simulink model "Speedgoat_Standalone_Sim_Dyno"  (R2021a)
settings: Solver=FixedStepDiscrete  StartTime=0.0  StopTime=inf  FixedStep=ModelTs  RelTol=1e-3
PreLoadFcn:
  | clc;
  | clear;
  | addpath ../
  | addpath(genpath('../../../settings/ParametersFiles/'))
  | addpath(genpath('../../../source/simulink/'))
  | BusInit;
  | filename_motor='';
  | filename_board='';
  | Thermal.Trotor = 25;
  | Thermal.Tstator = 25;
  | adc_out_mode = 1;  % 'ADC_voltage'  -- 0 --> 'ADC_counts'
  | InputCircuit.Vr = 230;  % ac voltage
  | ModelTs = 62.5e-6;  % 16KHz
undefined symbols (not defined in the file or in its folder): IO316, IO3xx, Motor
libraries: speedgoatlib_IO142 x3, speedgoatlib_fpga_pwm x3, simulink_extras x1, MapleSim_bpm_dq_dyno_xi_ie_16k_2018a x1, speedgoatlib_fpga x1
settings Model: SimulationMode=external  Creator=BEATOA  LastModifiedBy=lab.motori2
settings SolverCC: ConcurrentTasks=on  AlgebraicLoopSolver=TrustRegion  PositivePriorityOrder=on
settings DataIOCC: ReturnWorkspaceOutputs=off
settings OptimizationCC: BlockReduction=off  OptimizeBlockIOStorage=off
settings DebuggingCC: TasksWithSamePriorityMsg=none  SFMachineParentedDataDiag=warning  ArithmeticOperatorsInVariantConditions=warning
settings HardwareCC: ProdBitPerLong=64  ProdLongLongMode=on  ProdHWDeviceType=Intel->x86-64 (Linux 64)
settings SFSimCC: SimUseLocalCustomCode=off  CustomCodeUndefinedFunction=UseInterfaceOnly
settings RTWCC: Description=Simulink Real-Time  SystemTargetFile=slrealtime.tlc  TemplateMakefile=slrealtime_default_tmf  RTWUseLocalCustomCode=off  Toolchain=Simulink Real-Time Toolchain  BuildConfiguration=Faster Runs  CodeExecutionProfiling=on  TargetLang=C++

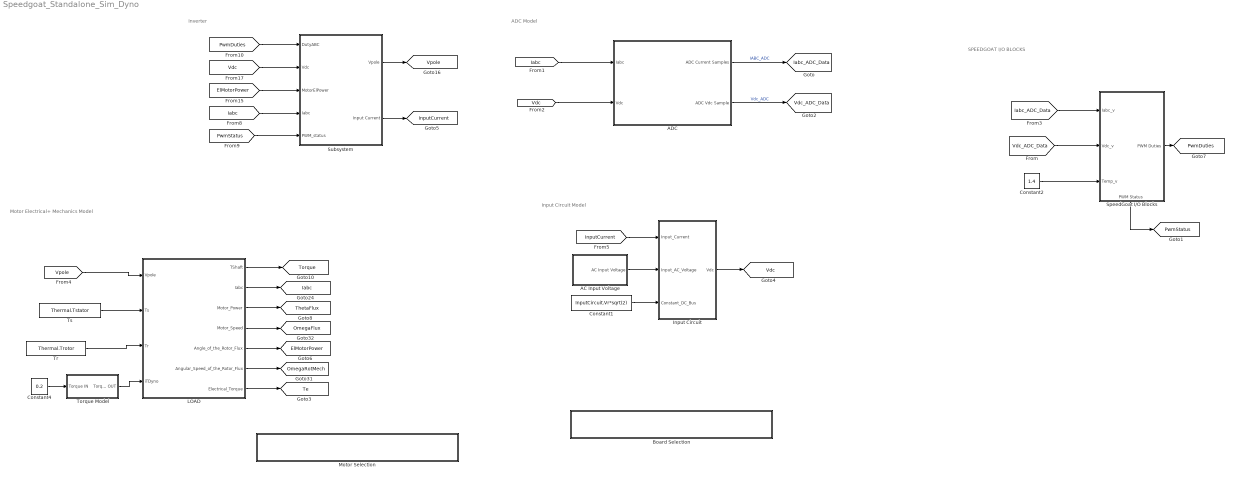
== system Speedgoat_Standalone_Sim_Dyno ==
  note: Inverter
  note: ADC Model
  note: Motor Electrical+ Mechanics Model
  note: SPEEDGOAT I/O BLOCKS
  note: Input Circuit Model
  AC Input Voltage : Subsystem
  ADC : Subsystem  mask{C1=InputCircuit.C1, C2=InputCircuit.C2, Cvolt=InputCircuit.Cvolt, ADCBit=InputCircuit.ADCBit, Vcc=InputCircuit.Vcc}
  Board Selection : Subsystem  TreatAsAtomicUnit=on  mask{ParamsFile=ColoradoPreliminary_AC230VPFC.xml}
      mask prompts: ParamsFile "Motor Parameters Selection"
      mask init:
      | myVal = evalin('base','filename_board');
      | set_param(gcb,'ParamsFile',myVal);
      settings: OpenFcn=|
      | filename_board = uigetfile({'*.xml'}, 'Select a board parameters File', ...
      |     '../../../settings/ParametersFiles/Rectifier_Parameters/');
      | run_rect_xml(filename_board);
      | set_param(gcb,'ParamsFile',filename_board);
      mask Display: disp(get_param(gcb,'ParamsFile'));
  Constant1 : Constant  Value=InputCircuit.Vr*sqrt(2)
  Constant2 : Constant  Value=1.4
  Constant4 : Constant  Value=0.2
  Input Circuit : Subsystem  Variant=on  VariantControlMode=label  VariantControl=Choice  LabelModeActiveChoice=Choice_2
  LOAD : Subsystem  Variant=on  VariantControlMode=label  LabelModeActiveChoice=Complete Motor
  Motor Selection : Subsystem  TreatAsAtomicUnit=on  mask{ParamsFile=BPM_Hefei_H27.xml}
      mask prompts: ParamsFile "Motor Parameters Selection"
      mask init:
      | myVal = evalin('base','filename_motor');
      | set_param(gcb,'ParamsFile',myVal);
      settings: OpenFcn=|
      | filename_motor = uigetfile({'*.xml'}, 'Select a motor parameters File', ...
      |     '../../../settings/ParametersFiles/Motor_Parameters/');
      | run_motor_bpm_xml(filename_motor);
      | set_param(gcb,'ParamsFile',filename_motor);
      mask Display: disp(get_param(gcb,'ParamsFile'));
  SpeedGoat I/O Blocks : Subsystem
      settings: PortSchema="{\"entries\":[{\"content\":{\"sides\":[{\"content\":{\"connectorIds\":[\"In1\",\"In2\",\"In3\"]},\"type\":\"ConnectorPlacement.EquallySpacedRectSide\",\"uuid\":\"6b9aa341-3ac4-4bf9-8aae-3ce5ce9c7d2d\"},{\"content\":{\"connectorIds\":[\"Out1\"],\"side\":\"RIGHT\"},\"type\":\"ConnectorPlacement.EquallySpacedRectSide\",\"uuid\":\"0e7969fa-09d9-4686-a5e1-30592a058991\"},{\"content\":{\"connectorIds\":[],\"side\":\"TOP\"},\"type\":\"ConnectorPlacement.EquallySpacedRectSide\",\"uuid\":\"94aad33f-2d4e-4106-b9bf-df6b0e16ba85\"},{\"content\":{\"connectorIds\":[\"Out2\"],\"side\":\"BOTTOM\"},\"type\":\"ConnectorPlacement.EquallySpacedRectSide\",\"uuid\":\"230b77cf-a16b-4a04-9d46-02ae57ab6957\"}]},\"type\":\"ConnectorPlacement.EquallySpacedConnector\",\"uuid\":\"7bdcd0a4-d700-4dbb-82d4-1eb3a47212ed\"}],\"packageUris\":[\"http://schema.mathworks.com/mf0/Connector/R2020b\"],\"version\":\"1.0\"}"
  Subsystem : Subsystem
  Torque Model : Subsystem
  Tr : Constant  Value=Thermal.Trotor
  Ts : Constant  Value=Thermal.Tstator
  tag scope: ElMotorPower=global, Iabc=global, Iabc_ADC_Data=global, InputCurrent=global, OmegaFlux=global, OmegaRotMech=global, PwmDuties=global, PwmStatus=global, Te=global, ThetaFlux=global, Torque=global, Vdc=global, Vdc_ADC_Data=global, Vpole=global
  wires:
  [Vdc] -> ADC/2(Vdc)
  ADC/1(ADC Current Samples) -> [Iabc_ADC_Data]  "IABC_ADC"
  ADC/2(ADC Vdc Sample) -> [Vdc_ADC_Data]  "Vdc_ADC"
  [Iabc] -> ADC/1(Iabc)
  [PwmDuties] -> Subsystem/1(DutyABC)
  [Vdc] -> Subsystem/2(Vdc)
  [ElMotorPower] -> Subsystem/3(MotorElPower)
  [Iabc] -> Subsystem/4(Iabc)
  [PwmStatus] -> Subsystem/5(PWM_status)
  Subsystem/1("Vpole ") -> [Vpole]
  Subsystem/2(Input Current) -> [InputCurrent]
  [Vpole] -> LOAD/1(Vpole)
  Ts/1 -> LOAD/2(Ts)
  Tr/1 -> LOAD/3(Tr)
  LOAD/1(TShaft) -> [Torque]
  LOAD/2(Iabc) -> [Iabc]
  LOAD/3(Motor_Power) -> [ThetaFlux]
  LOAD/4(Motor_Speed) -> [OmegaFlux]
  LOAD/5(Angle_of_the_Rotor_Flux) -> [ElMotorPower]
  LOAD/6(Angular_Speed_of_the_Rotor_Flux) -> [OmegaRotMech]
  LOAD/7(Electrical_Torque) -> [Te]
  Torque Model/1(Torque OUT) -> LOAD/4(iTDyno)
  [InputCurrent] -> Input Circuit/1(Input_Current)
  AC Input Voltage/1(AC Input Voltage) -> Input Circuit/2(Input_AC_Voltage)
  Constant1/1 -> Input Circuit/3(Constant_DC_Bus)
  Input Circuit/1(Vdc) -> [Vdc]
  [Iabc_ADC_Data] -> SpeedGoat I/O Blocks/1(Iabc_v)
  [Vdc_ADC_Data] -> SpeedGoat I/O Blocks/2(Vdc_v)
  SpeedGoat I/O Blocks/1(PWM Duties) -> [PwmDuties]
  Constant2/1 -> SpeedGoat I/O Blocks/3(Temp_v)
  Constant4/1 -> Torque Model/1(Torque IN)
  SpeedGoat I/O Blocks/2(PWM Status) -> [PwmStatus]

== system Speedgoat_Standalone_Sim_Dyno/AC Input Voltage ==
  Sine Wave : Sin  Amplitude=InputCircuit.Vr*sqrt(2)  Frequency=InputCircuit.freq*2*pi
  AC Input Voltage : Outport  VectorParamsAs1DForOutWhenUnconnected=off
  wires:
  Sine Wave/1 -> AC Input Voltage/1

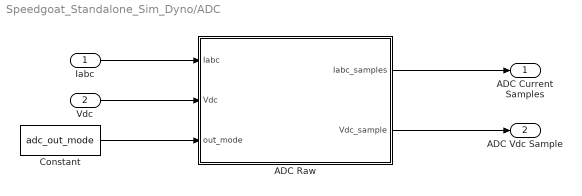
== system Speedgoat_Standalone_Sim_Dyno/ADC ==
  Iabc : Inport
  Vdc : Inport  Port=2
  ADC Raw : MATLAB Function  TreatAsAtomicUnit=on  mask{C1=C1, C2=C2, Cvolt=Cvolt, ADCBit=ADCBit, Vcc=Vcc}
      mask init:
      | C1=C1;
      | C2=C2;
      | Cvolt=Cvolt;
      | ADCBit=ADCBit;
      | Vcc=Vcc;
  Constant : Constant  Value=adc_out_mode
  ADC Current Samples : Outport  VectorParamsAs1DForOutWhenUnconnected=off
  ADC Vdc Sample : Outport  Port=2  VectorParamsAs1DForOutWhenUnconnected=off
  wires:
  Iabc/1 -> ADC Raw/1(Iabc)
  Vdc/1 -> ADC Raw/2(Vdc)
  ADC Raw/1(Iabc_samples) -> ADC Current Samples/1
  ADC Raw/2(Vdc_sample) -> ADC Vdc Sample/1
  Constant/1 -> ADC Raw/3(out_mode)

== system Speedgoat_Standalone_Sim_Dyno/Board Selection ==

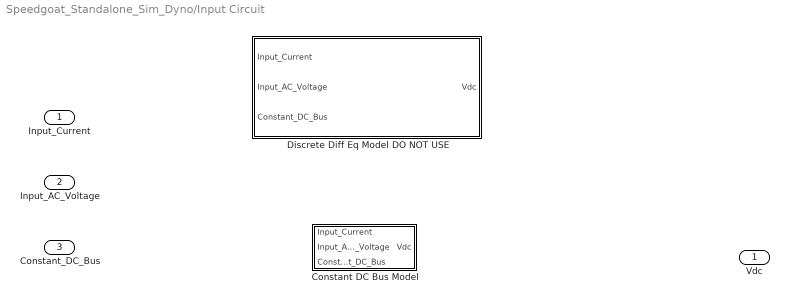
== system Speedgoat_Standalone_Sim_Dyno/Input Circuit ==
  Input_Current : Inport
  Input_AC_Voltage : Inport  Port=2
  Constant_DC_Bus : Inport  Port=3
  Constant DC Bus Model : Subsystem  TreatAsAtomicUnit=on  VariantControl=Choice_2
  Discrete Diff Eq Model DO NOT USE : MATLAB Function  TreatAsAtomicUnit=on  VariantControl=Choice_1  mask{tsample=ModelTs*4, C=InputCircuit.C_buscap, L=InputCircuit.L_line+InputCircuit.L_pfc, R=InputCircuit.R_line+InputCircuit.R_diode*2 +InputCircuit.R_pfc, Rinrush=6}
      mask prompts: C "Cbus"; L "Lin"; R "Rin"
  Vdc : Outport

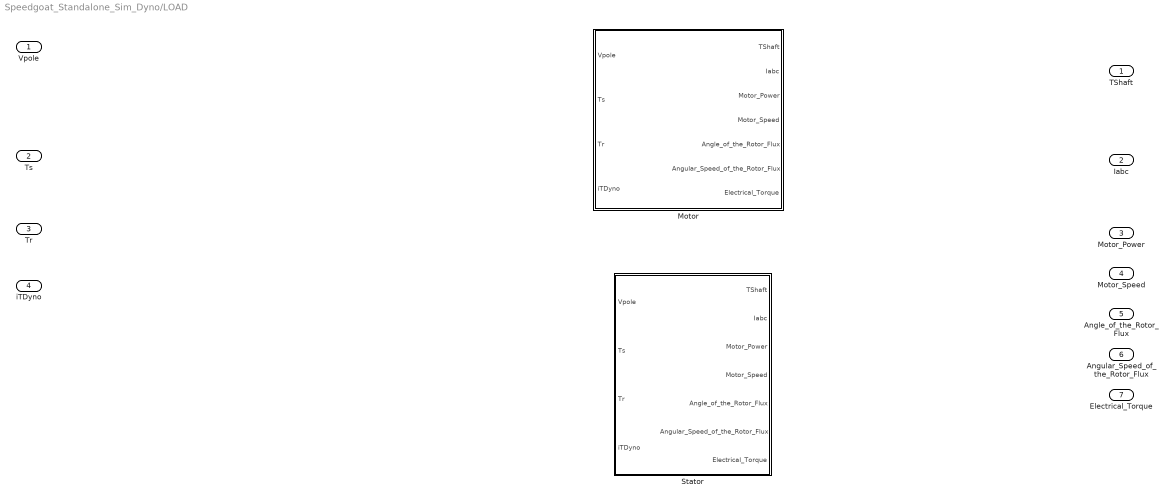
== system Speedgoat_Standalone_Sim_Dyno/LOAD ==
  Vpole : Inport
  Ts : Inport  Port=2
  Tr : Inport  Port=3
  iTDyno : Inport  Port=4
  Motor : Subsystem  VariantControl=Complete Motor
  Stator : Subsystem  VariantControl=Stator Only
  TShaft : Outport
  Iabc : Outport  Port=2
  Motor_Power : Outport  Port=3
  Motor_Speed : Outport  Port=4
  Angle_of_the_Rotor_Flux : Outport  Port=5
  Angular_Speed_of_the_Rotor_Flux : Outport  Port=6
  Electrical_Torque : Outport  Port=7

== system Speedgoat_Standalone_Sim_Dyno/Motor Selection ==

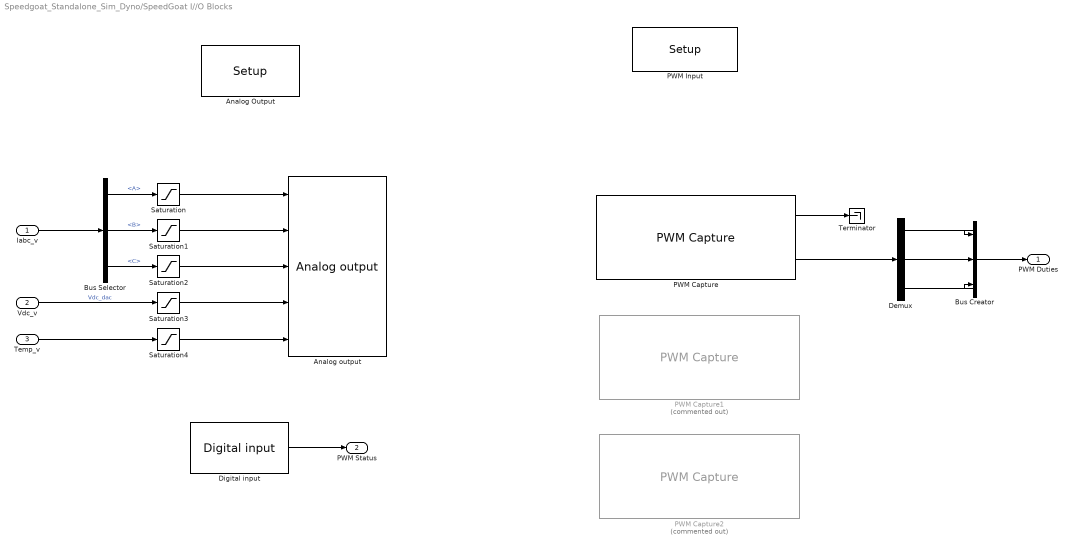
== system Speedgoat_Standalone_Sim_Dyno/SpeedGoat I//O Blocks ==
  Iabc_v : Inport
  Vdc_v : Inport  Port=2
  Temp_v : Inport  Port=3
  "Analog Output " : speedgoatlib_IO142/Setup   parPciSlot=-1  parModuleId=1  parInterModuleSync=Independent  parConvClockBaseRate=20MHz  parConvClock1Divider=20000  parConvClock2Divider=20000  parFrameTriggerEnable=off  parFrameTriggerDivider=10  parConvClock1BaseRate=1  parConvClock2BaseRate=1  parFrameTriggerClock=1  parAdcCoupling1=Differential  parAdcChannels1=[1 2]  parAdcChannel11=off  parAdcChannel12=off  parAdcChannel13=off  parAdcChannel14=off  parAdcChannel15=off  parAdcChannel16=off  parAdcChannel17=off  parAdcChannel18=off  parAdcRangeAll1=+-0.64 V  parVoltageRangePerChannelEn1=off  parAdcRange11=+-0.64 V  parAdcRange12=+-0.64 V  parAdcRange13=+-0.64 V  parAdcRange14=+-0.64 V  parAdcRange15=+-0.64 V  parAdcRange16=+-0.64 V  parAdcRange17=+-0.64 V  parAdcRange18=+-0.64 V  parAdcCoupling2=Differential  parAdcChannels2=[9 10]  parAdcChannel21=off  parAdcChannel22=off  parAdcChannel23=off  parAdcChannel24=off  parAdcChannel25=off  parAdcChannel26=off  parAdcChannel27=off  parAdcChannel28=off  parAdcRangeAll2=+-0.64 V  parVoltageRangePerChannelEn2=off  parAdcRange21=+-0.64 V  parAdcRange22=+-0.64 V  parAdcRange23=+-0.64 V  parAdcRange24=+-0.64 V  parAdcRange25=+-0.64 V  parAdcRange26=+-0.64 V  parAdcRange27=+-0.64 V  parAdcRange28=+-0.64 V  parAdcCoupling3=Differential  parAdcChannels3=[17 18]  parAdcChannel31=off  parAdcChannel32=off  parAdcChannel33=off  parAdcChannel34=off  parAdcChannel35=off  parAdcChannel36=off  parAdcChannel37=off  parAdcChannel38=off  parAdcRangeAll3=+-0.64 V  parVoltageRangePerChannelEn3=off  parAdcRange31=+-0.64 V  parAdcRange32=+-0.64 V  parAdcRange33=+-0.64 V  parAdcRange34=+-0.64 V  parAdcRange35=+-0.64 V  parAdcRange36=+-0.64 V  parAdcRange37=+-0.64 V  parAdcRange38=+-0.64 V  parAdcCoupling4=Differential  parAdcChannels4=[25 26]  parAdcChannel41=off  parAdcChannel42=off  parAdcChannel43=off  parAdcChannel44=off  parAdcChannel45=off  parAdcChannel46=off  parAdcChannel47=off  parAdcChannel48=off  parAdcRangeAll4=+-0.64 V  parVoltageRangePerChannelEn4=off  parAdcRange41=+-0.64 V  parAdcRange42=+-0.64 V  parAdcRange43=+-0.64 V  parAdcRange44=+-0.64 V  parAdcRange45=+-0.64 V  parAdcRange46=+-0.64 V  parAdcRange47=+-0.64 V  parAdcRange48=+-0.64 V  parAdcChannels=[]  parAdcNumActiveChannels=[0 0 0 0]  parAdcVoltageRange=[1 1 1 1 1 1 1 1 1 1 1 1 1 1 1 1 1 1 1 1 1 1 1 1 1 1 1 1 1 1 1 1]  parAdcCoupling=[1 1 1 1]  parAdcContSampling=off  parAdcAutoCorrection=on  parAdcDmaEnable=off  parAdcDmaClock=Clock 1  parAdcFrameSize_=100  parAdcSampleTime_=-1  parAdcActiveDmaDevices=[1 1 1 1]  parAdcFrameTriggerEnable=0  parAdcFrameSize=100  parAdcSampleTime=0.1  parDacChannels=[1 2 3 4]  parDacChannel1=on  parDacChannel2=on  parDacChannel3=on  parDacChannel4=on  parDacChannel5=on  parDacChannel6=off  parDacChannel7=off  parDacChannel8=off  parDacInitValues=0  parDacResets=1  parDacVoltageRange=[1 1 1 1 1 1 1 1]  parDacOverRange=[0 0 0 0 0 0 0 0]  parDacRange1=0-5 V  parDacInitValue1=0  parDacReset1=on  parDacRange2=0-5 V  parDacInitValue2=0  parDacReset2=on  parDacRange3=0-5 V  parDacInitValue3=0  parDacReset3=on  parDacRange4=0-5 V  parDacInitValue4=0  parDacReset4=on  parDacRange5=0-5 V  parDacInitValue5=0  parDacReset5=on  parDacRange6=0-5 V  parDacInitValue6=0  parDacReset6=on  parDacRange7=0-5 V  parDacInitValue7=0  parDacReset7=on  parDacRange8=0-5 V  parDacInitValue8=0  parDacReset8=on  parDacAutoCorrection=on  parDacSyncOut=on  parDacDmaEnable=off  parDacDmaLatency=Until next frame  parDacDmaClock=Clock 1  parDacFrameSize_=100  parDacSampleTime_=-1  parDacActiveDmaDevices=[1 1 1 1]  parDacFrameTriggerEnable=0  parDacFrameSize=100  parDacSampleTime=0.1  parDiChannels=1  parDoChannels=[2 3 4 5 6 7 8]  parDioChannel1=In  parDioChannel2=Out  parDioChannel3=Out  parDioChannel4=Out  parDioChannel5=Out  parDioChannel6=Out  parDioChannel7=Out  parDioChannel8=Out  parDoInitValues=[0 0 0 0 0 0 0]  parDoReset=[1 1 1 1 1 1 1]  parDoInitValue1=0  parDoReset1=on  parDoInitValue2=0  parDoReset2=on  parDoInitValue3=0  parDoReset3=on  parDoInitValue4=0  parDoReset4=on  parDoInitValue5=0  parDoReset5=on  parDoInitValue6=0  parDoReset6=on  parDoInitValue7=0  parDoReset7=on  parDoInitValue8=0  parDoReset8=on  parDiDebounceEnable=off  parDiDebounceTime=0  parDiDebounceValue=0  parDioPullRefFront=Pull-up 3.3 V  parDioPullRefRear=Floating
      settings: SourceProductName=Simulink Real-Time: Speedgoat I/O Blockset
  "Analog output " : speedgoatlib_IO142/Analog output   parModuleId=1  parSampleTime=-1  parPciSlot=-1  parDacChannels=[1 2 3 4 5]  parDacVoltageRange=[1 1 1 1 1 1 1 1]  parDacOverRange=[0 0 0 0 0 0 0 0]  parDacInitValues=[0 0 0 0 0]  parDacReset=[1 1 1 1 1]  parDacSyncOut=1  parDacDmaEnable=0  parDacActiveDmaDevices=[1 1 1 1]  parDacDmaLatency=2  parDacFrameSize=100
      settings: SourceProductName=Simulink Real-Time: Speedgoat I/O Blockset
  Bus Creator : BusCreator  Inputs=3  OutDataTypeStr=Bus: XabcBus
  Bus Selector : BusSelector  OutputSignals=A,B,C
  Demux : Demux  Outputs=3
  "Digital input " : speedgoatlib_IO142/Digital input   parModuleId=1  parSampleTime=-1  parPciSlot=-1  parDiChannels=1
      settings: SourceProductName=Simulink Real-Time: Speedgoat I/O Blockset
  PWM Capture : speedgoatlib_fpga_pwm/PWM Capture  id=1  chan=[8 9 10]  ts=-1  enableDma=on  pciSlot=-1  board=IO316-100k  captureMode=Use dedicated trigger input  bit_width_cap=24  captureTimeout_si=[0]  captureTimeout_eff=0  captureTimeout=[0]  debounce_si=10e-6  debounce_eff=10e-6  debounce=[750]  showHighDuration=off  showLowDuration=off  showPeriod=on  showDC16=on  showDC8=off  showTOn=off  showTOff=off  showValidData=off
      settings: SourceProductName=Simulink Real-Time: Speedgoat I/O Blockset
  PWM Capture1 : speedgoatlib_fpga_pwm/PWM Capture  Commented=on  id=1  chan=[9]  ts=-1  enableDma=on  pciSlot=-1  board=IO316-100k  captureMode=Use dedicated trigger input  bit_width_cap=24  captureTimeout_si=[0]  captureTimeout_eff=0  captureTimeout=[0]  debounce_si=10e-6  debounce_eff=10e-6  debounce=[750]  showHighDuration=off  showLowDuration=off  showPeriod=off  showDC16=on  showDC8=off  showTOn=off  showTOff=off  showValidData=off
      settings: SourceProductName=Simulink Real-Time: Speedgoat I/O Blockset
  PWM Capture2 : speedgoatlib_fpga_pwm/PWM Capture  Commented=on  id=1  chan=[10]  ts=-1  enableDma=on  pciSlot=-1  board=IO316-100k  captureMode=Use dedicated trigger input  bit_width_cap=24  captureTimeout_si=[0]  captureTimeout_eff=0  captureTimeout=[0]  debounce_si=10e-6  debounce_eff=10e-6  debounce=[750]  showHighDuration=off  showLowDuration=off  showPeriod=off  showDC16=on  showDC8=off  showTOn=off  showTOff=off  showValidData=off
      settings: SourceProductName=Simulink Real-Time: Speedgoat I/O Blockset
  PWM Input : speedgoatlib_fpga/Setup/Setup  board=IO316-100k  id=1  device_id=1  frontIO=None  rearIO=IO3xx-22  bitstreamFile=speedgoat_IO316_100k_22_CI_02387.mat  rev=1.0  timestamp_string=00/00/00 00:00:00  fpgaFreq=75 MHz  fpgaTick=13.33 ns  ProgSpiFlash=off  ProgBPIFlash=off  pciSlot=-1  PullRPort0=pull-up 3.3V  VioPort0=3.3V  PullRPort1=pull-up 3.3V  VioPort1=3.3V  PullRPort2=pull-up 3.3V  VioPort2=3.3V  PullRPort3=pull-up 3.3V  VioPort3=3.3V  PullRPort4=pull-up 3.3V  VioPort4=3.3V  PullRPort5=pull-up 3.3V  VioPort5=3.3V  PullRPort6=pull-up 3.3V  VioPort6=3.3V  PullRPort15=pull-up 3.3V  PullRPort31=pull-up 3.3V  PullRPort47=pull-up 3.3V  PullRPort63=pull-up 3.3V
      settings: SourceProductName=Simulink Real-Time: Speedgoat I/O Blockset
  Saturation{,1..4} (5 alike) : Saturate  UpperLimit=InputCircuit.Vcc  LowerLimit=0
  Terminator : Terminator
  PWM Duties : Outport
  PWM Status : Outport  Port=2
  wires:
  PWM Capture/1 -> Terminator/1
  Bus Selector/1 -> Saturation/1  "<A>"
  Bus Selector/3 -> Saturation2/1  "<C>"
  Vdc_v/1 -> Saturation3/1  "Vdc_dac"
  Temp_v/1 -> Saturation4/1
  Bus Selector/2 -> Saturation1/1  "<B>"
  Iabc_v/1 -> Bus Selector/1
  Bus Creator/1 -> PWM Duties/1
  Saturation/1 -> "Analog output "/1
  Saturation1/1 -> "Analog output "/2
  Saturation2/1 -> "Analog output "/3
  Saturation3/1 -> "Analog output "/4
  Saturation4/1 -> "Analog output "/5
  "Digital input "/1 -> PWM Status/1
  PWM Capture/2 -> Demux/1
  Demux/1 -> Bus Creator/1
  Demux/2 -> Bus Creator/2
  Demux/3 -> Bus Creator/3

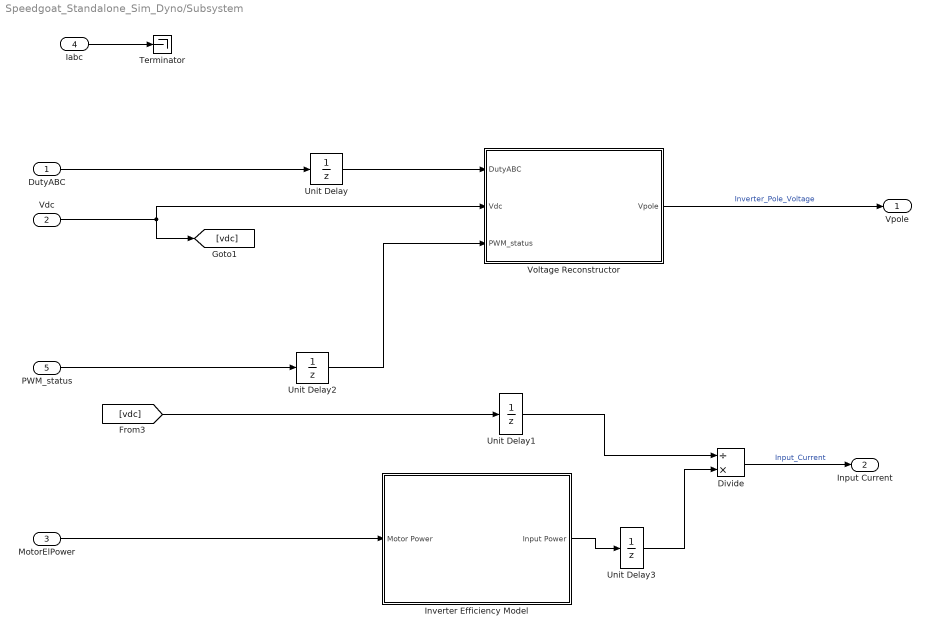
== system Speedgoat_Standalone_Sim_Dyno/Subsystem ==
  DutyABC : Inport  OutDataTypeStr=Bus: XabcBus
  Vdc : Inport  Port=2
  MotorElPower : Inport  Port=3
  Iabc : Inport  Port=4  OutDataTypeStr=Bus: XabcBus
  PWM_status : Inport  Port=5
  Divide : Product  Inputs=/*
  Inverter Efficiency Model : Subsystem
  Terminator : Terminator
  Unit Delay : UnitDelay  SampleTime=-1  HasFrameUpgradeWarning=on
  Unit Delay1 : UnitDelay  InitialCondition=InputCircuit.Vdc_i  SampleTime=-1  HasFrameUpgradeWarning=on
  Unit Delay2 : UnitDelay  SampleTime=-1  HasFrameUpgradeWarning=on
  Unit Delay3 : UnitDelay  SampleTime=-1  HasFrameUpgradeWarning=on
  Voltage Reconstructor : MATLAB Function  TreatAsAtomicUnit=on
  "Vpole " : Outport  OutDataTypeStr=Bus: XabcBus  VectorParamsAs1DForOutWhenUnconnected=off
  Input Current : Outport  Port=2  VectorParamsAs1DForOutWhenUnconnected=off
  wires:
  PWM_status/1 -> Unit Delay2/1
  Unit Delay3/1 -> Divide/2
  Unit Delay1/1 -> Divide/1
  Vdc/1 -> Voltage Reconstructor/2(Vdc), [vdc]
  Divide/1 -> Input Current/1  "Input_Current"
  Voltage Reconstructor/1(Vpole) -> "Vpole "/1  "Inverter_Pole_Voltage"
  Unit Delay/1 -> Voltage Reconstructor/1(DutyABC)
  Inverter Efficiency Model/1(Input Power) -> Unit Delay3/1
  Unit Delay2/1 -> Voltage Reconstructor/3(PWM_status)
  MotorElPower/1 -> Inverter Efficiency Model/1(Motor Power)
  DutyABC/1 -> Unit Delay/1
  [vdc] -> Unit Delay1/1
  Iabc/1 -> Terminator/1

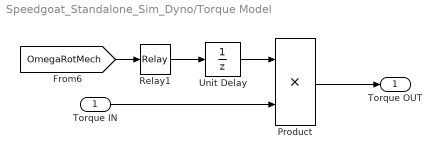
== system Speedgoat_Standalone_Sim_Dyno/Torque Model ==
  Torque IN : Inport
  Product : Product
  Relay1 : Relay  OnSwitchValue=300/60*6.28  OffSwitchValue=300/60*6.28
  Unit Delay : UnitDelay  SampleTime=-1  HasFrameUpgradeWarning=on
  Torque OUT : Outport
  wires:
  Product/1 -> Torque OUT/1
  [OmegaRotMech] -> Relay1/1
  Relay1/1 -> Unit Delay/1
  Torque IN/1 -> Product/2
  Unit Delay/1 -> Product/1

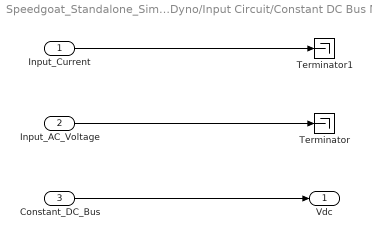
== system Speedgoat_Standalone_Sim_Dyno/Input Circuit/Constant DC Bus Model ==
  Input_Current : Inport
  Input_AC_Voltage : Inport  Port=2
  Constant_DC_Bus : Inport  Port=3
  Terminator : Terminator
  Terminator1 : Terminator
  Vdc : Outport
  wires:
  Input_AC_Voltage/1 -> Terminator/1
  Input_Current/1 -> Terminator1/1
  Constant_DC_Bus/1 -> Vdc/1

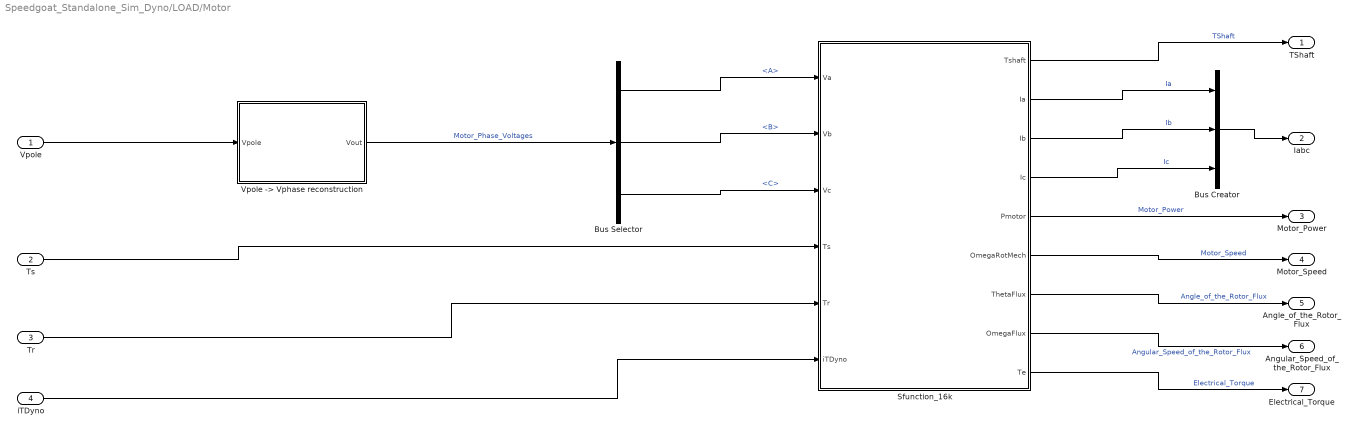
== system Speedgoat_Standalone_Sim_Dyno/LOAD/Motor ==
  Vpole : Inport
  Ts : Inport  Port=2
  Tr : Inport  Port=3
  iTDyno : Inport  Port=4
  Bus Creator : BusCreator  Inputs=3
  Bus Selector : BusSelector  OutputSignals=A,B,C
  Sfunction_16k : Subsystem  VariantControl=Variant_Motor_Model_Executable == 2
  "Vpole -> Vphase reconstruction" : MATLAB Function  TreatAsAtomicUnit=on
  TShaft : Outport
  Iabc : Outport  Port=2
  Motor_Power : Outport  Port=3
  Motor_Speed : Outport  Port=4
  Angle_of_the_Rotor_Flux : Outport  Port=5
  Angular_Speed_of_the_Rotor_Flux : Outport  Port=6
  Electrical_Torque : Outport  Port=7
  wires:
  Sfunction_16k/6(OmegaRotMech) -> Motor_Speed/1  "Motor_Speed"
  Sfunction_16k/7(ThetaFlux) -> Angle_of_the_Rotor_Flux/1  "Angle_of_the_Rotor_Flux"
  Sfunction_16k/9(Te) -> Electrical_Torque/1  "Electrical_Torque"
  Sfunction_16k/8(OmegaFlux) -> Angular_Speed_of_the_Rotor_Flux/1  "Angular_Speed_of_the_Rotor_Flux"
  Sfunction_16k/1(Tshaft) -> TShaft/1  "TShaft"
  Vpole/1 -> "Vpole -> Vphase reconstruction"/1(Vpole)
  iTDyno/1 -> Sfunction_16k/6(iTDyno)
  Ts/1 -> Sfunction_16k/4(Ts)
  Tr/1 -> Sfunction_16k/5(Tr)
  Sfunction_16k/5(Pmotor) -> Motor_Power/1  "Motor_Power"
  Bus Selector/2 -> Sfunction_16k/2(Vb)  "<B>"
  Bus Creator/1 -> Iabc/1
  Sfunction_16k/3(Ib) -> Bus Creator/2  "Ib"
  "Vpole -> Vphase reconstruction"/1(Vout) -> Bus Selector/1  "Motor_Phase_Voltages"
  Sfunction_16k/4(Ic) -> Bus Creator/3  "Ic"
  Sfunction_16k/2(Ia) -> Bus Creator/1  "Ia"
  Bus Selector/3 -> Sfunction_16k/3(Vc)  "<C>"
  Bus Selector/1 -> Sfunction_16k/1(Va)  "<A>"

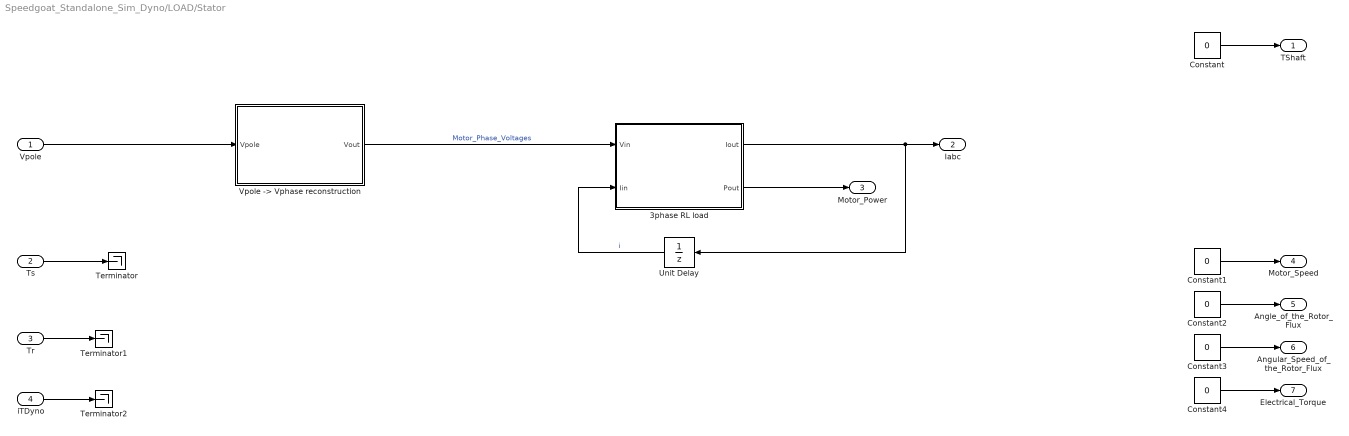
== system Speedgoat_Standalone_Sim_Dyno/LOAD/Stator ==
  Vpole : Inport
  Ts : Inport  Port=2
  Tr : Inport  Port=3
  iTDyno : Inport  Port=4
  3phase RL load : MATLAB Function  TreatAsAtomicUnit=on  mask{R=Motor.Electrical.Rs_a_Ref, L=Motor.Inductance_Variation.Ld_a0}
      mask prompts: R "Resistance"; L "Inductance"
  Constant{,1..4} (5 alike) : Constant  Value=0
  Terminator : Terminator
  Terminator1 : Terminator
  Terminator2 : Terminator
  Unit Delay : UnitDelay  SampleTime=-1  HasFrameUpgradeWarning=on
  "Vpole -> Vphase reconstruction" : MATLAB Function  TreatAsAtomicUnit=on
  TShaft : Outport
  Iabc : Outport  Port=2
  Motor_Power : Outport  Port=3
  Motor_Speed : Outport  Port=4
  Angle_of_the_Rotor_Flux : Outport  Port=5
  Angular_Speed_of_the_Rotor_Flux : Outport  Port=6
  Electrical_Torque : Outport  Port=7
  wires:
  "Vpole -> Vphase reconstruction"/1(Vout) -> 3phase RL load/1(Vin)  "Motor_Phase_Voltages"
  Vpole/1 -> "Vpole -> Vphase reconstruction"/1(Vpole)
  3phase RL load/1(Iout) -> Unit Delay/1, Iabc/1
  Unit Delay/1 -> 3phase RL load/2(Iin)  "i"
  Ts/1 -> Terminator/1
  Tr/1 -> Terminator1/1
  iTDyno/1 -> Terminator2/1
  Constant/1 -> TShaft/1
  Constant1/1 -> Motor_Speed/1
  Constant2/1 -> Angle_of_the_Rotor_Flux/1
  Constant3/1 -> Angular_Speed_of_the_Rotor_Flux/1
  Constant4/1 -> Electrical_Torque/1
  3phase RL load/2(Pout) -> Motor_Power/1

== system Speedgoat_Standalone_Sim_Dyno/Subsystem/Inverter Efficiency Model ==
  Motor Power : Inport
  Inverter Efficiency : Gain  Gain=1/1
  Input Power : Outport  VectorParamsAs1DForOutWhenUnconnected=off
  wires:
  Motor Power/1 -> Inverter Efficiency/1
  Inverter Efficiency/1 -> Input Power/1

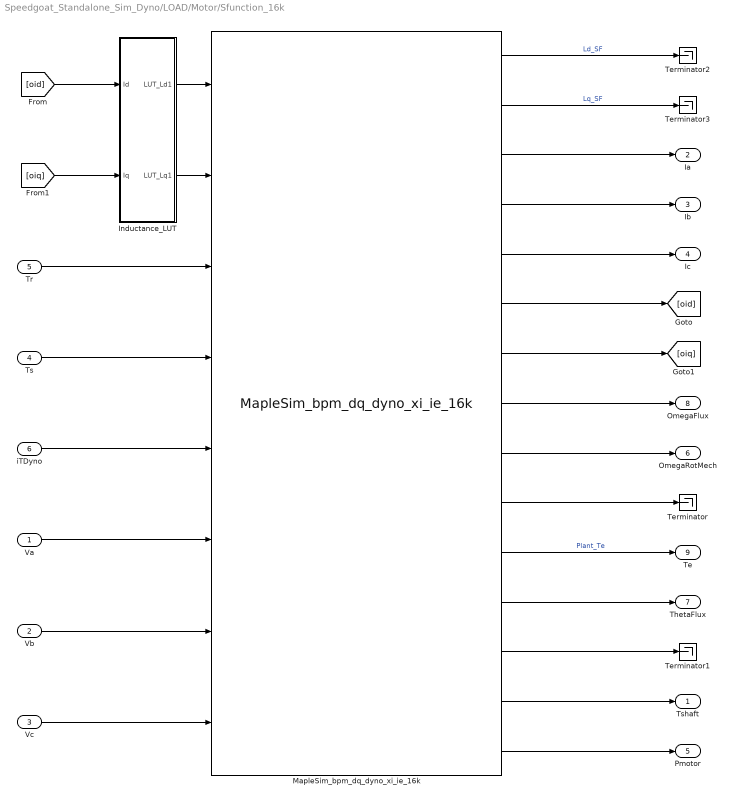
== system Speedgoat_Standalone_Sim_Dyno/LOAD/Motor/Sfunction_16k ==
  Va : Inport
  Vb : Inport  Port=2
  Vc : Inport  Port=3
  Ts : Inport  Port=4
  Tr : Inport  Port=5
  iTDyno : Inport  Port=6
  Inductance_LUT : Subsystem
  MapleSim_bpm_dq_dyno_xi_ie_16k : MapleSim_bpm_dq_dyno_xi_ie_16k_2018a/MapleSim_bpm_dq_dyno_xi_ie_16k  Description=Subsystem: MapleSim_bpm_dq_dyno_xi_ie_16k  ic=[0., 0., 0., 0.]  Par1=Motor.Mechanical.B  Par2=Motor.Mechanical.Jrotor  Par3=Motor.Inductance_Variation.Ld_a0  Par4=Motor.Inductance_Variation.Lq_b0  Par5=Motor.Electrical.p_Pole_Pairs  Par6=Motor.Electrical.Rs_a_Ref  Par7=Motor.Mechanical.PM_Temperature_Ref  Par8=Motor.Mechanical.Rs_Temperature_Ref  Par9=Motor.Electrical.alpha_s  Par10=.206e-2  Par11=Motor.Electrical.PM_Flux_f01  MinStep=1/40
  Terminator{,1..3} (4 alike) : Terminator
  Tshaft : Outport  VectorParamsAs1DForOutWhenUnconnected=off
  Ia : Outport  Port=2  VectorParamsAs1DForOutWhenUnconnected=off
  Ib : Outport  Port=3  VectorParamsAs1DForOutWhenUnconnected=off
  Ic : Outport  Port=4  VectorParamsAs1DForOutWhenUnconnected=off
  Pmotor : Outport  Port=5  VectorParamsAs1DForOutWhenUnconnected=off
  OmegaRotMech : Outport  Port=6  VectorParamsAs1DForOutWhenUnconnected=off
  ThetaFlux : Outport  Port=7  VectorParamsAs1DForOutWhenUnconnected=off
  OmegaFlux : Outport  Port=8  VectorParamsAs1DForOutWhenUnconnected=off
  Te : Outport  Port=9  VectorParamsAs1DForOutWhenUnconnected=off
  wires:
  MapleSim_bpm_dq_dyno_xi_ie_16k/5 -> Ic/1
  MapleSim_bpm_dq_dyno_xi_ie_16k/12 -> ThetaFlux/1
  iTDyno/1 -> MapleSim_bpm_dq_dyno_xi_ie_16k/5
  Vc/1 -> MapleSim_bpm_dq_dyno_xi_ie_16k/8
  MapleSim_bpm_dq_dyno_xi_ie_16k/15 -> Pmotor/1
  MapleSim_bpm_dq_dyno_xi_ie_16k/8 -> OmegaFlux/1
  MapleSim_bpm_dq_dyno_xi_ie_16k/14 -> Tshaft/1
  Vb/1 -> MapleSim_bpm_dq_dyno_xi_ie_16k/7
  MapleSim_bpm_dq_dyno_xi_ie_16k/9 -> OmegaRotMech/1
  MapleSim_bpm_dq_dyno_xi_ie_16k/4 -> Ib/1
  MapleSim_bpm_dq_dyno_xi_ie_16k/11 -> Te/1  "Plant_Te"
  Ts/1 -> MapleSim_bpm_dq_dyno_xi_ie_16k/4
  MapleSim_bpm_dq_dyno_xi_ie_16k/3 -> Ia/1
  Va/1 -> MapleSim_bpm_dq_dyno_xi_ie_16k/6
  Tr/1 -> MapleSim_bpm_dq_dyno_xi_ie_16k/3
  MapleSim_bpm_dq_dyno_xi_ie_16k/10 -> Terminator/1
  MapleSim_bpm_dq_dyno_xi_ie_16k/13 -> Terminator1/1
  [oiq] -> Inductance_LUT/2(Iq)
  [oid] -> Inductance_LUT/1(Id)
  Inductance_LUT/2(LUT_Lq1) -> MapleSim_bpm_dq_dyno_xi_ie_16k/2
  Inductance_LUT/1(LUT_Ld1) -> MapleSim_bpm_dq_dyno_xi_ie_16k/1
  MapleSim_bpm_dq_dyno_xi_ie_16k/1 -> Terminator2/1  "Ld_SF"
  MapleSim_bpm_dq_dyno_xi_ie_16k/2 -> Terminator3/1  "Lq_SF"
  MapleSim_bpm_dq_dyno_xi_ie_16k/6 -> [oid]
  MapleSim_bpm_dq_dyno_xi_ie_16k/7 -> [oiq]

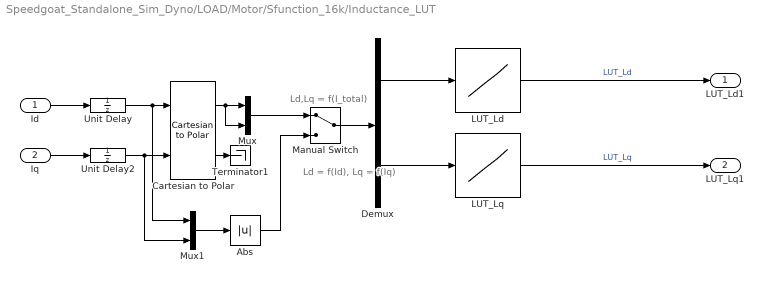
== system Speedgoat_Standalone_Sim_Dyno/LOAD/Motor/Sfunction_16k/Inductance_LUT ==
  note: Ld,Lq = f(I_total)
  note: Ld = f(Id),
      | Lq = f(Iq)
  Id : Inport
  Iq : Inport  Port=2
  Abs : Abs
  Cartesian to Polar : simulink_extras/Transformations/Cartesian to Polar
  Demux : Demux  Outputs=2
  LUT_Ld : Lookup_n-D  NumberOfTableDimensions=1  BreakpointsForDimension1=[Motor.Inductance_Variation.I_pk0,Motor.Inductance_Variation.I_pk1,Motor.Inductance_Variation.I_pk2,Motor.Inductance_Variation.I_pk3,Motor.Inductance_Variation.I_pk4,Motor.Inductance_Variation.I_pk5,Motor.Inductance_Variation.I_pk6,Motor.Inductance_Variation.I_pk7]  IndexSearchMethod=Evenly spaced points  Table=[Motor.Inductance_Variation.Ld_a0,Motor.Inductance_Variation.Ld_a1,Motor.Inductance_Variation.Ld_a2,Motor.Inductance_Variation.Ld_a3,Motor.Inductance_Variation.Ld_a4,Motor.Inductance_Variation.Ld_a5,Motor.Inductance_Variation.Ld_a6,Motor.Inductance_Variation.Ld_a7]  InternalRulePriority=Speed  RndMeth=Simplest  InputSameDT=on
  LUT_Lq : Lookup_n-D  NumberOfTableDimensions=1  BreakpointsForDimension1=[Motor.Inductance_Variation.I_pk0,Motor.Inductance_Variation.I_pk1,Motor.Inductance_Variation.I_pk2,Motor.Inductance_Variation.I_pk3,Motor.Inductance_Variation.I_pk4,Motor.Inductance_Variation.I_pk5,Motor.Inductance_Variation.I_pk6,Motor.Inductance_Variation.I_pk7]  IndexSearchMethod=Evenly spaced points  Table=[Motor.Inductance_Variation.Lq_b0,Motor.Inductance_Variation.Lq_b1,Motor.Inductance_Variation.Lq_b2,Motor.Inductance_Variation.Lq_b3,Motor.Inductance_Variation.Lq_b4,Motor.Inductance_Variation.Lq_b5,Motor.Inductance_Variation.Lq_b6,Motor.Inductance_Variation.Lq_b7]  InternalRulePriority=Speed  RndMeth=Simplest  InputSameDT=on
  Manual Switch : ManualSwitch
  Mux : Mux  Inputs=2
  Mux1 : Mux  Inputs=2
  Terminator1 : Terminator
  Unit Delay : UnitDelay  SampleTime=-1  HasFrameUpgradeWarning=on
  Unit Delay2 : UnitDelay  SampleTime=-1  HasFrameUpgradeWarning=on
  LUT_Ld1 : Outport  VectorParamsAs1DForOutWhenUnconnected=off
  LUT_Lq1 : Outport  Port=2  VectorParamsAs1DForOutWhenUnconnected=off
  wires:
  LUT_Ld/1 -> LUT_Ld1/1  "LUT_Ld"
  Cartesian to Polar/1 -> Mux/2, Mux/1
  Unit Delay/1 -> Mux1/1, Cartesian to Polar/1
  Unit Delay2/1 -> Mux1/2, Cartesian to Polar/2
  Mux/1 -> Manual Switch/1
  Demux/1 -> LUT_Ld/1
  Iq/1 -> Unit Delay2/1
  Cartesian to Polar/2 -> Terminator1/1
  Manual Switch/1 -> Demux/1
  Mux1/1 -> Abs/1
  Demux/2 -> LUT_Lq/1
  LUT_Lq/1 -> LUT_Lq1/1  "LUT_Lq"
  Id/1 -> Unit Delay/1
  Abs/1 -> Manual Switch/2

== matlab function Speedgoat_Standalone_Sim_Dyno/LOAD/Stator/3phase RL load ==
  data: Vin input Bus: XabcBus; Iout output Bus: XabcBus; Iin input Bus: XabcBus; L parameter; R parameter; ModelTs parameter; Pout output
function [Iout,Pout]   = RL_TF(Vin,Iin, L, R, ModelTs)


Iout.A = (1-R*ModelTs/L)*Iin.A + Vin.A*ModelTs/L;
Iout.B = (1-R*ModelTs/L)*Iin.B + Vin.B*ModelTs/L;
Iout.C = (1-R*ModelTs/L)*Iin.C + Vin.C*ModelTs/L;

Pout = Iin.A*Vin.A + Iin.B*Vin.B + Iin.C*Vin.C;
end

== matlab function Speedgoat_Standalone_Sim_Dyno/Input Circuit/Discrete Diff Eq Model DO NOT USE ==
  data: Input_Current input; Vdc output double size=1; Input_AC_Voltage input double size=1; Constant_DC_Bus input; tsample parameter double size=1; L parameter double size=1; R parameter double size=1; C parameter double size=1; Rinrush parameter double size=1
function Vdc = Rect_Simple(Input_Current, Input_AC_Voltage, Constant_DC_Bus, tsample,L, R, C,Rinrush)
if Input_Current == 0
    iout = 0.05;
else
    iout = Input_Current;
end
Vac = Input_AC_Voltage;
persistent iout_1;
persistent vdc_1;
persistent vdc_2;
persistent state;
persistent inrush;
if isempty(iout_1)
    iout_1 = 0;
end
if isempty(vdc_1)
    vdc_1 = 200;
end
if isempty(vdc_2)
    vdc_2 = 200;
end
if isempty(state)
    state = -1;  %first switch-on
end
if isempty(inrush)
    inrush = 1;
end


%tsample = 62.5e-6;
%Rinrush = 6;
%C = 330e-6;
%L = 0.0097 + 0.00005;
Rin = R + inrush* Rinrush;
% if (Vdc_1 < 50)
%     iout = 0;
% else
%     iout = Pin/Vdc_1;
% end
%Pin = iout *Vdc_1;
%omega_2 = 1/L/C;
%k = R/(2*L);
%beta = sqrt(omega_2-k^2);

alpha = L*C + Rin*C*tsample;
a1 = tsample^2 - 2*L*C - Rin*C*tsample;
a2 = L*C;
a3 = L*tsample;
a4 = L* tsample - Rin*tsample^2;
a5 = tsample^2;

Vin = abs(Vac);


if state == 0%Vdc_1 >= Vin
    %arg = Vdc_1^2 - 2/C * tsample * Pin;
    %if arg >= 0
        %Vdc = sqrt(Vdc_1^2 - 2/C * tsample * Pin); 
        Vdc = vdc_1 - 1/C * tsample * iout; 
    %else
    %    Vdc = 0;
    %end
    iL = 0;
else

    %https://www.dam.brown.edu/people/alcyew/handouts/numdiff.pdf
    Vdc  = 1/alpha * (-a1*vdc_1-a2*vdc_2-a3*iout+a4*iout_1+a5*Vin);
    iL = iout + C/tsample * (Vdc - vdc_1);
end
vdc_2 = vdc_1;
vdc_1 = Vdc;
iout_1 = iout;

if (state == 0)
     if (Vin>=vdc_1)
         state = 1;
     end
elseif (state == 1)
     %if (Vin<vdc_1)
     if (iL <0)
         state = 0;
         inrush = 0;
     end
elseif  (state == -1)
    state = 1;
    inrush = 1;
end

== matlab function Speedgoat_Standalone_Sim_Dyno/LOAD/Motor/Vpole -> Vphase reconstruction ==
  data: Vpole input Bus: XabcBus size=1; Vout output Bus: XabcBus
function Vout   = Vrec2(Vpole)

Va = Vpole.A;
Vb = Vpole.B;
Vc = Vpole.C;

Vn = (Va + Vb + Vc)/3;

Vphase.A = Va - Vn;
Vphase.B = Vb - Vn;
Vphase.C = Vc - Vn;

Vline.A = Va - Vb;  % Vab
Vline.B = Vb - Vc;  % Vbc
Vline.C = Vc - Va;  % Vca

Vout = Vphase;
end

== matlab function Speedgoat_Standalone_Sim_Dyno/LOAD/Stator/Vpole -> Vphase reconstruction ==
  data: Vpole input Bus: XabcBus size=1; Vout output Bus: XabcBus
function Vout   = Vrec2(Vpole)

Va = Vpole.A;
Vb = Vpole.B;
Vc = Vpole.C;

Vn = (Va + Vb + Vc)/3;

Vphase.A = Va - Vn;
Vphase.B = Vb - Vn;
Vphase.C = Vc - Vn;

Vline.A = Va - Vb;  % Vab
Vline.B = Vb - Vc;  % Vbc
Vline.C = Vc - Va;  % Vca

Vout = Vphase;
end

== matlab function Speedgoat_Standalone_Sim_Dyno/Subsystem/Voltage Reconstructor ==
  data: DutyABC input Bus: XabcBus size=1; Vpole output Bus: XabcBus size=1; Vdc input; PWM_status input
function Vpole   = Vrec(DutyABC, Vdc, PWM_status)

if (PWM_status == 1)
    Da = DutyABC.A;
    Db = DutyABC.B;
    Dc = DutyABC.C;
else
    Da = 0.5;
    Db = 0.5;
    Dc = 0.5;
end
Vpole.A = Vdc * Da;
Vpole.B = Vdc * Db;
Vpole.C = Vdc * Dc;

== matlab function Speedgoat_Standalone_Sim_Dyno/ADC/ADC Raw ==
  data: Iabc input Bus: XabcBus; Iabc_samples output Bus: XabcBus; Vdc input; Vdc_sample output; C1 parameter; C2 parameter; Cvolt parameter; Vcc parameter; ADCBit parameter; out_mode input
function [Iabc_samples, Vdc_sample] = GetADCRawData(Iabc,Vdc, C1, C2, Cvolt, Vcc, ADCBit,out_mode)
%#codegen
% out_mode == 0 --> ADC_counts
% out_mode == 1 --> ADC_voltage
% other --> out = 0

Iabc_samples.A = GetIRaw(Iabc.A,C1,C2,ADCBit, Vcc,out_mode);
Iabc_samples.B = GetIRaw(Iabc.B,C1,C2,ADCBit,Vcc,out_mode); 
Iabc_samples.C = GetIRaw(Iabc.C,C1,C2,ADCBit,Vcc,out_mode); 

Vdc_sample = GetVdcRaw(Vdc,Cvolt,ADCBit,Vcc,out_mode);
end



function vo = GetIRaw(I,C1,C2,ADCBit,Vcc, out_mode)
Vout=C1*I+C2;
if(Vout>Vcc)
    Vout=Vcc;
elseif (Vout<0)
    Vout=0;
end
if out_mode == 0        % ADC_counts
    vo=round((Vout/Vcc)*2^ADCBit);
elseif out_mode == 1    % ADC_voltage
    vo=Vout;
else 
    vo = 0;
end
end

function vo = GetVdcRaw(Vdc,Cvolt,ADCBit,Vcc,out_mode)
Vout=Cvolt*Vdc;
if(Vout>Vcc)
    Vout=Vcc;
elseif (Vout<0)
    Vout=0;
end
if out_mode == 0        % ADC_counts
    vo=round((Vout/Vcc)*2^ADCBit);
elseif out_mode == 1    % ADC_voltage
    vo=Vout;
else 
    vo = 0;
end
end
